simulink library "LibEEPROM_eeprom_example_ORIGINAL"  (Simulink 10.0)
settings: Solver=VariableStepAuto  StartTime=0.0  StopTime=10.0  RelTol=1e-3
undefined symbols (not defined in the file): CRC32_calc_and_EEPROM_Write_ALL, crc32_calc_intern, CRC32_EEPROM_Read, EEPROM_Mirror, EEPROM_Read, IO_Blk_Lib_TTC500, IO_EEPROM_GetStatus, IO_EEPROM_Init, IO_EEPROM_Write, Read_Mirror, Write_Mirror, Write_Mirror_prepare_EEPROM
libraries: simulink x56
(part 6 of 8)

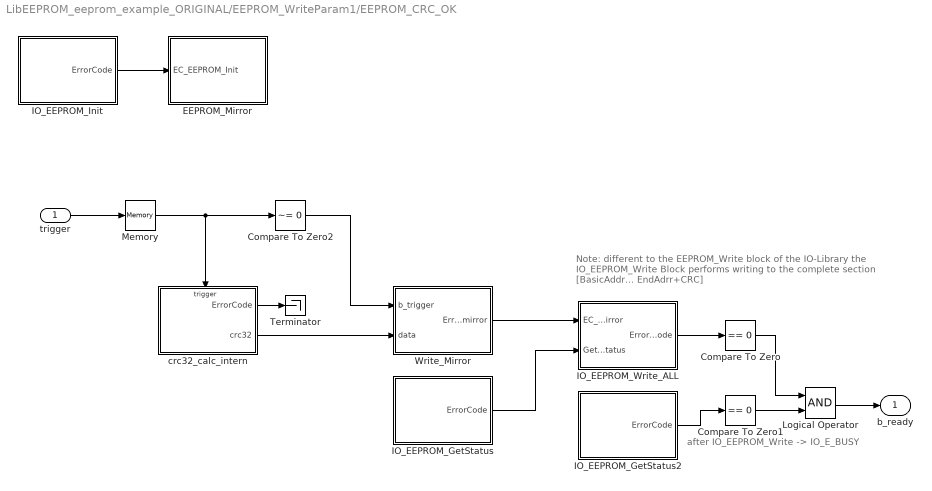
== system LibEEPROM_eeprom_example_ORIGINAL/EEPROM_WriteParam1/EEPROM_CRC_OK ==
  note: Note: different to the EEPROM_Write block
      | of the IO-Library the IO_EEPROM_Write Block
      | performs writing to the complete section [BasicAddr... EndAdrr+CRC]
  note: after IO_EEPROM_Write -> IO_E_BUSY
  trigger : Inport
  Compare To Zero : simulink/Logic and Bit Operations/Compare To Zero  relop===  OutDataTypeStr=boolean  ZeroCross=off
  Compare To Zero1 : simulink/Logic and Bit Operations/Compare To Zero  relop===  OutDataTypeStr=boolean  ZeroCross=off
  Compare To Zero2 : simulink/Logic and Bit Operations/Compare To Zero  relop=~=  OutDataTypeStr=boolean  ZeroCross=off
  EEPROM_Mirror : Subsystem  LoadFcn=|  mask(EEPROM_Mirror_Code){SampleTime=-1, ttlib=IO_Blk_Lib_TTC500, ttDescription=EEPROM_Mirror, tt_iolib_version=0.21, offset=0, length=65536}
      | try
      | %
      | %Upgrade Information - standard BEGIN
      | new_color = 'blue';
      | new_ver = '0.21';
      | act_ver = get_param(gcb,'tt_iolib_version');
      | if not(strcmp(act_ver,new_ver))
      |     disp(['Upgrade block: ',gcb,char(10),'       Version: ',act_ver,' -> ',new_ver]);
      |     %switch - case for specific upgrade information e.g. additional parameter required 
      |     %Change appearance and version information
      |     set_param(gcb,'ForegroundColor',new_color);
      |     set_param(gcb,'tt_iolib_version',new_ver);
      | end
      | %Upgrade Information - standard END
      | catch
      | %Standard catch section BEGIN 
      | disp(' ');
      | disp('------------------------------------------------------------');
      | disp('An error occurred in a callback of the TTC580-BlockLib.');
      | disp(['Please check the parameters in the mask of ',gcb]);
      | disp('If you do not encounter any violations, then please '); 
      | disp('copy the following lines and report this to support@ttcontrol.com ');
      | disp('<< begin of error message dump >>');
      | disp(['Version of TTC580-BlockLib: ', get_param(gcb,'tt_iolib_version')]);
      | disp(get_param(gcb,'ttDescription'));
      | disp(gcb);
      | x=lasterror;disp(x.message);
      | disp(get_param(gcb,'MaskValues'));
      | disp(version);
      | disp(computer);
      | disp('<< end of error message dump >>');
      | disp('------------------------------------------------------------');
      | disp(' ');
      | %Standard catch section END
      | end
      mask help:
      | Read all data from the EEPROM and mirror this onto RAM.
      | The ErrorCode of IO_EEPROM_Init - block must be connected to the input of EEPROM_Mirror.
      | After calling EEPROM_Mirror the global variable EEPROM_mirror is filled and
      | the global variable ErrorCode_EEPROM_mirror contains the returns of IO_EEPROM_Init() and IO_EEPROM_Read().
      mask init:
      | %
      settings: CopyFcn=%deleted
      mask Help: web(which('IO_EEPROM.h'))
      mask Callback offset: %
      mask Callback length: %
  IO_EEPROM_GetStatus : Subsystem  LoadFcn=|  mask(IO_EEPROM_GetStatus_Code){SampleTime=-1, ttlib=IO_Blk_Lib_TTC500, ttDescription=IO_EEPROM_GetStatus, tt_iolib_version=0.19}
      | try
      | %
      | %Upgrade Information - standard BEGIN
      | new_color = 'blue';
      | new_ver = '0.19';
      | act_ver = get_param(gcb,'tt_iolib_version');
      | if not(strcmp(act_ver,new_ver))
      |     disp(['Upgrade block: ',gcb,char(10),'       Version: ',act_ver,' -> ',new_ver]);
      |     %switch - case for specific upgrade information e.g. additional parameter required 
      |     %Change appearance and version information
      |     set_param(gcb,'ForegroundColor',new_color);
      |     set_param(gcb,'tt_iolib_version',new_ver);
      | end
      | %Upgrade Information - standard END
      | catch
      | %Standard catch section BEGIN 
      | disp(' ');
      | disp('------------------------------------------------------------');
      | disp('An error occurred in a callback of the TTC580-BlockLib.');
      | disp('Please copy the following lines and report this to support@tttech.com ');
      | disp('<< begin of error message dump >>');
      | disp(['Version of TTC580-BlockLib: ', get_param(gcb,'tt_iolib_version')]);
      | disp(get_param(gcb,'ttDescription'));
      | disp(gcb);
      | x=lasterror;disp(x.message);
      | disp(get_param(gcb,'MaskValues'));
      | disp(version);
      | disp(computer);
      | disp('<< end of error message dump >>');
      | disp('------------------------------------------------------------');
      | disp(' ');
      | %Standard catch section END
      | end
      mask help: Returns the status of the EEPROM driver.
      mask init:
      | %
      settings: CopyFcn=%deleted
      mask Help: web(which('IO_EEPROM.h'))
  IO_EEPROM_GetStatus2 : Subsystem  LoadFcn=|  mask(IO_EEPROM_GetStatus_Code){SampleTime=-1, ttlib=IO_Blk_Lib_TTC500, ttDescription=IO_EEPROM_GetStatus, tt_iolib_version=0.19}
      | try
      | %
      | %Upgrade Information - standard BEGIN
      | new_color = 'blue';
      | new_ver = '0.19';
      | act_ver = get_param(gcb,'tt_iolib_version');
      | if not(strcmp(act_ver,new_ver))
      |     disp(['Upgrade block: ',gcb,char(10),'       Version: ',act_ver,' -> ',new_ver]);
      |     %switch - case for specific upgrade information e.g. additional parameter required 
      |     %Change appearance and version information
      |     set_param(gcb,'ForegroundColor',new_color);
      |     set_param(gcb,'tt_iolib_version',new_ver);
      | end
      | %Upgrade Information - standard END
      | catch
      | %Standard catch section BEGIN 
      | disp(' ');
      | disp('------------------------------------------------------------');
      | disp('An error occurred in a callback of the TTC580-BlockLib.');
      | disp('Please copy the following lines and report this to support@tttech.com ');
      | disp('<< begin of error message dump >>');
      | disp(['Version of TTC580-BlockLib: ', get_param(gcb,'tt_iolib_version')]);
      | disp(get_param(gcb,'ttDescription'));
      | disp(gcb);
      | x=lasterror;disp(x.message);
      | disp(get_param(gcb,'MaskValues'));
      | disp(version);
      | disp(computer);
      | disp('<< end of error message dump >>');
      | disp('------------------------------------------------------------');
      | disp(' ');
      | %Standard catch section END
      | end
      mask help: Returns the status of the EEPROM driver.
      mask init:
      | %
      settings: CopyFcn=%deleted
      mask Help: web(which('IO_EEPROM.h'))
  IO_EEPROM_Init : Subsystem  LoadFcn=|  mask(IO_EEPROM_Init_Code){SampleTime=-1, ttlib=IO_Blk_Lib_TTC500, ttDescription=IO_EEPROM_Init, tt_iolib_version=0.19}
      | try
      | %
      | %Upgrade Information - standard BEGIN
      | new_color = 'blue';
      | new_ver = '0.19';
      | act_ver = get_param(gcb,'tt_iolib_version');
      | if not(strcmp(act_ver,new_ver))
      |     disp(['Upgrade block: ',gcb,char(10),'       Version: ',act_ver,' -> ',new_ver]);
      |     %switch - case for specific upgrade information e.g. additional parameter required 
      |     %Change appearance and version information
      |     set_param(gcb,'ForegroundColor',new_color);
      |     set_param(gcb,'tt_iolib_version',new_ver);
      | end
      | %Upgrade Information - standard END
      | catch
      | %Standard catch section BEGIN 
      | disp(' ');
      | disp('------------------------------------------------------------');
      | disp('An error occurred in a callback of the TTC580-BlockLib.');
      | disp('Please copy the following lines and report this to support@tttech.com ');
      | disp('<< begin of error message dump >>');
      | disp(['Version of TTC580-BlockLib: ', get_param(gcb,'tt_iolib_version')]);
      | disp(get_param(gcb,'ttDescription'));
      | disp(gcb);
      | x=lasterror;disp(x.message);
      | disp(get_param(gcb,'MaskValues'));
      | disp(version);
      | disp(computer);
      | disp('<< end of error message dump >>');
      | disp('------------------------------------------------------------');
      | disp(' ');
      | %Standard catch section END
      | end
      mask help: Initialization of the EEPROM driver.
      mask init:
      | %
      settings: CopyFcn=%deleted
      mask Help: web(which('IO_EEPROM.h'))
  IO_EEPROM_Write_ALL : Subsystem  LoadFcn=|  mask(IO_EEPROM_Write_Code){SampleTime=-1, ttlib=IO_Blk_Lib_TTC500, ttDescription=IO_EEPROM_Write, tt_iolib_version=0.19, offset=BasicAddr, length=EndAddr-BasicAddr+1+length}
      | try
      | %
      | %Upgrade Information - standard BEGIN
      | new_color = 'blue';
      | new_ver = '0.19';
      | act_ver = get_param(gcb,'tt_iolib_version');
      | if not(strcmp(act_ver,new_ver))
      |     disp(['Upgrade block: ',gcb,char(10),'       Version: ',act_ver,' -> ',new_ver]);
      |     %switch - case for specific upgrade information e.g. additional parameter required 
      |     %Change appearance and version information
      |     set_param(gcb,'ForegroundColor',new_color);
      |     set_param(gcb,'tt_iolib_version',new_ver);
      | end
      | %Upgrade Information - standard END
      | catch
      | %Standard catch section BEGIN 
      | disp(' ');
      | disp('------------------------------------------------------------');
      | disp('An error occurred in a callback of the TTC580-BlockLib.');
      | disp('Please copy the following lines and report this to support@tttech.com ');
      | disp('<< begin of error message dump >>');
      | disp(['Version of TTC580-BlockLib: ', get_param(gcb,'tt_iolib_version')]);
      | disp(get_param(gcb,'ttDescription'));
      | disp(gcb);
      | x=lasterror;disp(x.message);
      | disp(get_param(gcb,'MaskValues'));
      | disp(version);
      | disp(computer);
      | disp('<< end of error message dump >>');
      | disp('------------------------------------------------------------');
      | disp(' ');
      | %Standard catch section END
      | end
      mask help:
      | Copy data from EEPROM_mirror[] to physical EEPROM. Copy activity is triggered by the edge of the input "EC_Write_Mirror" from IO_E_BUSY to IO_E_OK.
      | The output "ErrorCode" is IO_E_BUSY as long as writing to EEPROM is pending. During the activities are performed writing to the physical EEPROM, "ErrorCode" corresponds to the output of the C-driver IO_EEPROM_Write().
      mask init:
      | %
      settings: CopyFcn=%deleted
      mask Help: web(which('IO_EEPROM.h'))
      mask Callback offset: %
      mask Callback length: %
  Logical Operator : Logic  AllPortsSameDT=off  OutDataTypeStr=boolean
  Memory : Memory  LinearizeAsDelay=on
  Terminator : Terminator
  Write_Mirror : Subsystem  LoadFcn=|  mask(Write_Mirror_Code){SampleTime=-1, ttlib=IO_Blk_Lib_TTC500, ttDescription=Write_Mirror, tt_iolib_version=0.19, offset=offset, length=length}
      | try
      | %
      | %Upgrade Information - standard BEGIN
      | new_color = 'blue';
      | new_ver = '0.19';
      | act_ver = get_param(gcb,'tt_iolib_version');
      | if not(strcmp(act_ver,new_ver))
      |     disp(['Upgrade block: ',gcb,char(10),'       Version: ',act_ver,' -> ',new_ver]);
      |     %switch - case for specific upgrade information e.g. additional parameter required 
      |     %Change appearance and version information
      |     set_param(gcb,'ForegroundColor',new_color);
      |     set_param(gcb,'tt_iolib_version',new_ver);
      | end
      | %Upgrade Information - standard END
      | catch
      | %Standard catch section BEGIN 
      | disp(' ');
      | disp('------------------------------------------------------------');
      | disp('An error occurred in a callback of the TTC580-BlockLib.');
      | disp('Please copy the following lines and report this to support@tttech.com ');
      | disp('<< begin of error message dump >>');
      | disp(['Version of TTC580-BlockLib: ', get_param(gcb,'tt_iolib_version')]);
      | disp(get_param(gcb,'ttDescription'));
      | disp(gcb);
      | x=lasterror;disp(x.message);
      | disp(get_param(gcb,'MaskValues'));
      | disp(version);
      | disp(computer);
      | disp('<< end of error message dump >>');
      | disp('------------------------------------------------------------');
      | disp(' ');
      | %Standard catch section END
      | end
      mask help:
      | Write data to the mirror of the EEPROM. ErrorCode is set to IO_E_BUSY for one cycle of writing into EEPROM_mirror[].
      | In case the given data section exceeds given EEPROM boundaries, IO_E_EEPROM_RANGE ErrorCode is returned.
      mask init:
      | %
      settings: CopyFcn=%deleted
      mask Help: web(which('~.h'))
      mask Callback offset: %
      mask Callback length: %
  crc32_calc_intern : Subsystem  LoadFcn=|  mask(crc32_calc_intern_Code){SampleTime=-1, ttlib=IO_Blk_Lib_TTC500, ttDescription=crc32_calc_intern, tt_iolib_version=0.19, EEPROM_mirror=EEPROM_mirror, iBasicAddr_intern=BasicAddr, iEndAddr_intern=EndAddr}
      | try
      | %
      | %Upgrade Information - standard BEGIN
      | new_color = 'blue';
      | new_ver = '0.19';
      | act_ver = get_param(gcb,'tt_iolib_version');
      | if not(strcmp(act_ver,new_ver))
      |     disp(['Upgrade block: ',gcb,char(10),'       Version: ',act_ver,' -> ',new_ver]);
      |     %switch - case for specific upgrade information e.g. additional parameter required 
      |     %Change appearance and version information
      |     set_param(gcb,'ForegroundColor',new_color);
      |     set_param(gcb,'tt_iolib_version',new_ver);
      | end
      | %Upgrade Information - standard END
      | catch
      | %Standard catch section BEGIN 
      | disp(' ');
      | disp('------------------------------------------------------------');
      | disp('An error occurred in a callback of the TTC580-BlockLib.');
      | disp('Please copy the following lines and report this to support@tttech.com ');
      | disp('<< begin of error message dump >>');
      | disp(['Version of TTC580-BlockLib: ', get_param(gcb,'tt_iolib_version')]);
      | disp(get_param(gcb,'ttDescription'));
      | disp(gcb);
      | x=lasterror;disp(x.message);
      | disp(get_param(gcb,'MaskValues'));
      | disp(version);
      | disp(computer);
      | disp('<< end of error message dump >>');
      | disp('------------------------------------------------------------');
      | disp(' ');
      | %Standard catch section END
      | end
      mask help:
      | Calculate crc32 for a section out of the EEPROM.
      | In case the given data section exceeds given EEPROM boundaries, non zero ErrorCode is returned.
      mask init:
      | %
      settings: CopyFcn=%deleted
      mask Help: No further help available for this block
      mask Callback EEPROM_mirror: %
      mask Callback iBasicAddr_intern: %
      mask Callback iEndAddr_intern: %
  b_ready : Outport  VectorParamsAs1DForOutWhenUnconnected=off
  wires:
  Compare To Zero1/1 -> Logical Operator/2
  crc32_calc_intern/1(ErrorCode) -> Terminator/1
  Logical Operator/1 -> b_ready/1
  Compare To Zero/1 -> Logical Operator/1
  Memory/1 -> Compare To Zero2/1, crc32_calc_intern/Trigger
  Compare To Zero2/1 -> Write_Mirror/1(b_trigger)
  crc32_calc_intern/2(crc32) -> Write_Mirror/2(data)
  IO_EEPROM_GetStatus/1(ErrorCode) -> IO_EEPROM_Write_ALL/2(GetStatus)
  Write_Mirror/1(ErrorCode_EEPROM_mirror) -> IO_EEPROM_Write_ALL/1(EC_Write_Mirror)
  trigger/1 -> Memory/1
  IO_EEPROM_Write_ALL/1(ErrorCode) -> Compare To Zero/1
  IO_EEPROM_Init/1(ErrorCode) -> EEPROM_Mirror/1(EC_EEPROM_Init)
  IO_EEPROM_GetStatus2/1(ErrorCode) -> Compare To Zero1/1

== system LibEEPROM_eeprom_example_ORIGINAL/EEPROM_WriteParam1/EEPROM_param_1 ==
  note: NO IO_EEPROM_Write
      | perfomted here. This is
      | done in CRC32_calc_and_EEPROM_Write_ALL
  trigger : Inport
  data : Inport  Port=2  OutDataTypeStr=EEPROM_type
  Compare To Zero : simulink/Logic and Bit Operations/Compare To Zero  relop===  OutDataTypeStr=boolean  ZeroCross=off
  Compare To Zero1 : simulink/Logic and Bit Operations/Compare To Zero  relop=~=  OutDataTypeStr=boolean  ZeroCross=off
  Write_Mirror : Subsystem  LoadFcn=|  mask(Write_Mirror_Code){SampleTime=-1, ttlib=IO_Blk_Lib_TTC500, ttDescription=Write_Mirror, tt_iolib_version=0.19, offset=offset, length=length}
      | try
      | %
      | %Upgrade Information - standard BEGIN
      | new_color = 'blue';
      | new_ver = '0.19';
      | act_ver = get_param(gcb,'tt_iolib_version');
      | if not(strcmp(act_ver,new_ver))
      |     disp(['Upgrade block: ',gcb,char(10),'       Version: ',act_ver,' -> ',new_ver]);
      |     %switch - case for specific upgrade information e.g. additional parameter required 
      |     %Change appearance and version information
      |     set_param(gcb,'ForegroundColor',new_color);
      |     set_param(gcb,'tt_iolib_version',new_ver);
      | end
      | %Upgrade Information - standard END
      | catch
      | %Standard catch section BEGIN 
      | disp(' ');
      | disp('------------------------------------------------------------');
      | disp('An error occurred in a callback of the TTC580-BlockLib.');
      | disp('Please copy the following lines and report this to support@tttech.com ');
      | disp('<< begin of error message dump >>');
      | disp(['Version of TTC580-BlockLib: ', get_param(gcb,'tt_iolib_version')]);
      | disp(get_param(gcb,'ttDescription'));
      | disp(gcb);
      | x=lasterror;disp(x.message);
      | disp(get_param(gcb,'MaskValues'));
      | disp(version);
      | disp(computer);
      | disp('<< end of error message dump >>');
      | disp('------------------------------------------------------------');
      | disp(' ');
      | %Standard catch section END
      | end
      mask help:
      | Write data to the mirror of the EEPROM. ErrorCode is set to IO_E_BUSY for one cycle of writing into EEPROM_mirror[].
      | In case the given data section exceeds given EEPROM boundaries, IO_E_EEPROM_RANGE ErrorCode is returned.
      mask init:
      | %
      settings: CopyFcn=%deleted
      mask Help: web(which('~.h'))
      mask Callback offset: %
      mask Callback length: %
  b_ready : Outport  VectorParamsAs1DForOutWhenUnconnected=off
  wires:
  Compare To Zero1/1 -> Write_Mirror/1(b_trigger)
  Write_Mirror/1(ErrorCode_EEPROM_mirror) -> Compare To Zero/1
  data/1 -> Write_Mirror/2(data)
  trigger/1 -> Compare To Zero1/1
  Compare To Zero/1 -> b_ready/1

== system LibEEPROM_eeprom_example_ORIGINAL/EEPROM_WriteParam1/EEPROM_param_2 ==
  note: NO IO_EEPROM_Write
      | perfomted here. This is
      | done in CRC32_calc_and_EEPROM_Write_ALL
  trigger : Inport
  data : Inport  Port=2  OutDataTypeStr=EEPROM_type
  Compare To Zero : simulink/Logic and Bit Operations/Compare To Zero  relop===  OutDataTypeStr=boolean  ZeroCross=off
  Compare To Zero1 : simulink/Logic and Bit Operations/Compare To Zero  relop=~=  OutDataTypeStr=boolean  ZeroCross=off
  Write_Mirror : Subsystem  LoadFcn=|  mask(Write_Mirror_Code){SampleTime=-1, ttlib=IO_Blk_Lib_TTC500, ttDescription=Write_Mirror, tt_iolib_version=0.19, offset=offset, length=length}
      | try
      | %
      | %Upgrade Information - standard BEGIN
      | new_color = 'blue';
      | new_ver = '0.19';
      | act_ver = get_param(gcb,'tt_iolib_version');
      | if not(strcmp(act_ver,new_ver))
      |     disp(['Upgrade block: ',gcb,char(10),'       Version: ',act_ver,' -> ',new_ver]);
      |     %switch - case for specific upgrade information e.g. additional parameter required 
      |     %Change appearance and version information
      |     set_param(gcb,'ForegroundColor',new_color);
      |     set_param(gcb,'tt_iolib_version',new_ver);
      | end
      | %Upgrade Information - standard END
      | catch
      | %Standard catch section BEGIN 
      | disp(' ');
      | disp('------------------------------------------------------------');
      | disp('An error occurred in a callback of the TTC580-BlockLib.');
      | disp('Please copy the following lines and report this to support@tttech.com ');
      | disp('<< begin of error message dump >>');
      | disp(['Version of TTC580-BlockLib: ', get_param(gcb,'tt_iolib_version')]);
      | disp(get_param(gcb,'ttDescription'));
      | disp(gcb);
      | x=lasterror;disp(x.message);
      | disp(get_param(gcb,'MaskValues'));
      | disp(version);
      | disp(computer);
      | disp('<< end of error message dump >>');
      | disp('------------------------------------------------------------');
      | disp(' ');
      | %Standard catch section END
      | end
      mask help:
      | Write data to the mirror of the EEPROM. ErrorCode is set to IO_E_BUSY for one cycle of writing into EEPROM_mirror[].
      | In case the given data section exceeds given EEPROM boundaries, IO_E_EEPROM_RANGE ErrorCode is returned.
      mask init:
      | %
      settings: CopyFcn=%deleted
      mask Help: web(which('~.h'))
      mask Callback offset: %
      mask Callback length: %
  b_ready : Outport  VectorParamsAs1DForOutWhenUnconnected=off
  wires:
  Compare To Zero1/1 -> Write_Mirror/1(b_trigger)
  Write_Mirror/1(ErrorCode_EEPROM_mirror) -> Compare To Zero/1
  data/1 -> Write_Mirror/2(data)
  trigger/1 -> Compare To Zero1/1
  Compare To Zero/1 -> b_ready/1

== system LibEEPROM_eeprom_example_ORIGINAL/EEPROM_WriteParam1/EEPROM_param_3 ==
  note: NO IO_EEPROM_Write
      | perfomted here. This is
      | done in CRC32_calc_and_EEPROM_Write_ALL
  trigger : Inport
  data : Inport  Port=2  OutDataTypeStr=EEPROM_type
  Compare To Zero : simulink/Logic and Bit Operations/Compare To Zero  relop===  OutDataTypeStr=boolean  ZeroCross=off
  Compare To Zero1 : simulink/Logic and Bit Operations/Compare To Zero  relop=~=  OutDataTypeStr=boolean  ZeroCross=off
  Write_Mirror : Subsystem  LoadFcn=|  mask(Write_Mirror_Code){SampleTime=-1, ttlib=IO_Blk_Lib_TTC500, ttDescription=Write_Mirror, tt_iolib_version=0.19, offset=offset, length=length}
      | try
      | %
      | %Upgrade Information - standard BEGIN
      | new_color = 'blue';
      | new_ver = '0.19';
      | act_ver = get_param(gcb,'tt_iolib_version');
      | if not(strcmp(act_ver,new_ver))
      |     disp(['Upgrade block: ',gcb,char(10),'       Version: ',act_ver,' -> ',new_ver]);
      |     %switch - case for specific upgrade information e.g. additional parameter required 
      |     %Change appearance and version information
      |     set_param(gcb,'ForegroundColor',new_color);
      |     set_param(gcb,'tt_iolib_version',new_ver);
      | end
      | %Upgrade Information - standard END
      | catch
      | %Standard catch section BEGIN 
      | disp(' ');
      | disp('------------------------------------------------------------');
      | disp('An error occurred in a callback of the TTC580-BlockLib.');
      | disp('Please copy the following lines and report this to support@tttech.com ');
      | disp('<< begin of error message dump >>');
      | disp(['Version of TTC580-BlockLib: ', get_param(gcb,'tt_iolib_version')]);
      | disp(get_param(gcb,'ttDescription'));
      | disp(gcb);
      | x=lasterror;disp(x.message);
      | disp(get_param(gcb,'MaskValues'));
      | disp(version);
      | disp(computer);
      | disp('<< end of error message dump >>');
      | disp('------------------------------------------------------------');
      | disp(' ');
      | %Standard catch section END
      | end
      mask help:
      | Write data to the mirror of the EEPROM. ErrorCode is set to IO_E_BUSY for one cycle of writing into EEPROM_mirror[].
      | In case the given data section exceeds given EEPROM boundaries, IO_E_EEPROM_RANGE ErrorCode is returned.
      mask init:
      | %
      settings: CopyFcn=%deleted
      mask Help: web(which('~.h'))
      mask Callback offset: %
      mask Callback length: %
  b_ready : Outport  VectorParamsAs1DForOutWhenUnconnected=off
  wires:
  Compare To Zero1/1 -> Write_Mirror/1(b_trigger)
  Write_Mirror/1(ErrorCode_EEPROM_mirror) -> Compare To Zero/1
  data/1 -> Write_Mirror/2(data)
  trigger/1 -> Compare To Zero1/1
  Compare To Zero/1 -> b_ready/1

== system LibEEPROM_eeprom_example_ORIGINAL/EEPROM_WriteParam1/EEPROM_param_4 ==
  note: NO IO_EEPROM_Write
      | perfomted here. This is
      | done in CRC32_calc_and_EEPROM_Write_ALL
  trigger : Inport
  data : Inport  Port=2  OutDataTypeStr=EEPROM_type
  Compare To Zero : simulink/Logic and Bit Operations/Compare To Zero  relop===  OutDataTypeStr=boolean  ZeroCross=off
  Compare To Zero1 : simulink/Logic and Bit Operations/Compare To Zero  relop=~=  OutDataTypeStr=boolean  ZeroCross=off
  Write_Mirror : Subsystem  LoadFcn=|  mask(Write_Mirror_Code){SampleTime=-1, ttlib=IO_Blk_Lib_TTC500, ttDescription=Write_Mirror, tt_iolib_version=0.19, offset=offset, length=length}
      | try
      | %
      | %Upgrade Information - standard BEGIN
      | new_color = 'blue';
      | new_ver = '0.19';
      | act_ver = get_param(gcb,'tt_iolib_version');
      | if not(strcmp(act_ver,new_ver))
      |     disp(['Upgrade block: ',gcb,char(10),'       Version: ',act_ver,' -> ',new_ver]);
      |     %switch - case for specific upgrade information e.g. additional parameter required 
      |     %Change appearance and version information
      |     set_param(gcb,'ForegroundColor',new_color);
      |     set_param(gcb,'tt_iolib_version',new_ver);
      | end
      | %Upgrade Information - standard END
      | catch
      | %Standard catch section BEGIN 
      | disp(' ');
      | disp('------------------------------------------------------------');
      | disp('An error occurred in a callback of the TTC580-BlockLib.');
      | disp('Please copy the following lines and report this to support@tttech.com ');
      | disp('<< begin of error message dump >>');
      | disp(['Version of TTC580-BlockLib: ', get_param(gcb,'tt_iolib_version')]);
      | disp(get_param(gcb,'ttDescription'));
      | disp(gcb);
      | x=lasterror;disp(x.message);
      | disp(get_param(gcb,'MaskValues'));
      | disp(version);
      | disp(computer);
      | disp('<< end of error message dump >>');
      | disp('------------------------------------------------------------');
      | disp(' ');
      | %Standard catch section END
      | end
      mask help:
      | Write data to the mirror of the EEPROM. ErrorCode is set to IO_E_BUSY for one cycle of writing into EEPROM_mirror[].
      | In case the given data section exceeds given EEPROM boundaries, IO_E_EEPROM_RANGE ErrorCode is returned.
      mask init:
      | %
      settings: CopyFcn=%deleted
      mask Help: web(which('~.h'))
      mask Callback offset: %
      mask Callback length: %
  b_ready : Outport  VectorParamsAs1DForOutWhenUnconnected=off
  wires:
  Compare To Zero1/1 -> Write_Mirror/1(b_trigger)
  Write_Mirror/1(ErrorCode_EEPROM_mirror) -> Compare To Zero/1
  data/1 -> Write_Mirror/2(data)
  trigger/1 -> Compare To Zero1/1
  Compare To Zero/1 -> b_ready/1

== system LibEEPROM_eeprom_example_ORIGINAL/EEPROM_WriteParam1/EEPROM_param_5 ==
  note: NO IO_EEPROM_Write
      | perfomted here. This is
      | done in CRC32_calc_and_EEPROM_Write_ALL
  trigger : Inport
  data : Inport  Port=2  OutDataTypeStr=EEPROM_type
  Compare To Zero : simulink/Logic and Bit Operations/Compare To Zero  relop===  OutDataTypeStr=boolean  ZeroCross=off
  Compare To Zero1 : simulink/Logic and Bit Operations/Compare To Zero  relop=~=  OutDataTypeStr=boolean  ZeroCross=off
  Write_Mirror : Subsystem  LoadFcn=|  mask(Write_Mirror_Code){SampleTime=-1, ttlib=IO_Blk_Lib_TTC500, ttDescription=Write_Mirror, tt_iolib_version=0.19, offset=offset, length=length}
      | try
      | %
      | %Upgrade Information - standard BEGIN
      | new_color = 'blue';
      | new_ver = '0.19';
      | act_ver = get_param(gcb,'tt_iolib_version');
      | if not(strcmp(act_ver,new_ver))
      |     disp(['Upgrade block: ',gcb,char(10),'       Version: ',act_ver,' -> ',new_ver]);
      |     %switch - case for specific upgrade information e.g. additional parameter required 
      |     %Change appearance and version information
      |     set_param(gcb,'ForegroundColor',new_color);
      |     set_param(gcb,'tt_iolib_version',new_ver);
      | end
      | %Upgrade Information - standard END
      | catch
      | %Standard catch section BEGIN 
      | disp(' ');
      | disp('------------------------------------------------------------');
      | disp('An error occurred in a callback of the TTC580-BlockLib.');
      | disp('Please copy the following lines and report this to support@tttech.com ');
      | disp('<< begin of error message dump >>');
      | disp(['Version of TTC580-BlockLib: ', get_param(gcb,'tt_iolib_version')]);
      | disp(get_param(gcb,'ttDescription'));
      | disp(gcb);
      | x=lasterror;disp(x.message);
      | disp(get_param(gcb,'MaskValues'));
      | disp(version);
      | disp(computer);
      | disp('<< end of error message dump >>');
      | disp('------------------------------------------------------------');
      | disp(' ');
      | %Standard catch section END
      | end
      mask help:
      | Write data to the mirror of the EEPROM. ErrorCode is set to IO_E_BUSY for one cycle of writing into EEPROM_mirror[].
      | In case the given data section exceeds given EEPROM boundaries, IO_E_EEPROM_RANGE ErrorCode is returned.
      mask init:
      | %
      settings: CopyFcn=%deleted
      mask Help: web(which('~.h'))
      mask Callback offset: %
      mask Callback length: %
  b_ready : Outport  VectorParamsAs1DForOutWhenUnconnected=off
  wires:
  Compare To Zero1/1 -> Write_Mirror/1(b_trigger)
  Write_Mirror/1(ErrorCode_EEPROM_mirror) -> Compare To Zero/1
  data/1 -> Write_Mirror/2(data)
  trigger/1 -> Compare To Zero1/1
  Compare To Zero/1 -> b_ready/1

== system LibEEPROM_eeprom_example_ORIGINAL/EEPROM_WriteParam1/EEPROM_param_6 ==
  note: NO IO_EEPROM_Write
      | perfomted here. This is
      | done in CRC32_calc_and_EEPROM_Write_ALL
  trigger : Inport
  data : Inport  Port=2  OutDataTypeStr=EEPROM_type
  Compare To Zero : simulink/Logic and Bit Operations/Compare To Zero  relop===  OutDataTypeStr=boolean  ZeroCross=off
  Compare To Zero1 : simulink/Logic and Bit Operations/Compare To Zero  relop=~=  OutDataTypeStr=boolean  ZeroCross=off
  Write_Mirror : Subsystem  LoadFcn=|  mask(Write_Mirror_Code){SampleTime=-1, ttlib=IO_Blk_Lib_TTC500, ttDescription=Write_Mirror, tt_iolib_version=0.19, offset=offset, length=length}
      | try
      | %
      | %Upgrade Information - standard BEGIN
      | new_color = 'blue';
      | new_ver = '0.19';
      | act_ver = get_param(gcb,'tt_iolib_version');
      | if not(strcmp(act_ver,new_ver))
      |     disp(['Upgrade block: ',gcb,char(10),'       Version: ',act_ver,' -> ',new_ver]);
      |     %switch - case for specific upgrade information e.g. additional parameter required 
      |     %Change appearance and version information
      |     set_param(gcb,'ForegroundColor',new_color);
      |     set_param(gcb,'tt_iolib_version',new_ver);
      | end
      | %Upgrade Information - standard END
      | catch
      | %Standard catch section BEGIN 
      | disp(' ');
      | disp('------------------------------------------------------------');
      | disp('An error occurred in a callback of the TTC580-BlockLib.');
      | disp('Please copy the following lines and report this to support@tttech.com ');
      | disp('<< begin of error message dump >>');
      | disp(['Version of TTC580-BlockLib: ', get_param(gcb,'tt_iolib_version')]);
      | disp(get_param(gcb,'ttDescription'));
      | disp(gcb);
      | x=lasterror;disp(x.message);
      | disp(get_param(gcb,'MaskValues'));
      | disp(version);
      | disp(computer);
      | disp('<< end of error message dump >>');
      | disp('------------------------------------------------------------');
      | disp(' ');
      | %Standard catch section END
      | end
      mask help:
      | Write data to the mirror of the EEPROM. ErrorCode is set to IO_E_BUSY for one cycle of writing into EEPROM_mirror[].
      | In case the given data section exceeds given EEPROM boundaries, IO_E_EEPROM_RANGE ErrorCode is returned.
      mask init:
      | %
      settings: CopyFcn=%deleted
      mask Help: web(which('~.h'))
      mask Callback offset: %
      mask Callback length: %
  b_ready : Outport  VectorParamsAs1DForOutWhenUnconnected=off
  wires:
  Compare To Zero1/1 -> Write_Mirror/1(b_trigger)
  Write_Mirror/1(ErrorCode_EEPROM_mirror) -> Compare To Zero/1
  data/1 -> Write_Mirror/2(data)
  trigger/1 -> Compare To Zero1/1
  Compare To Zero/1 -> b_ready/1

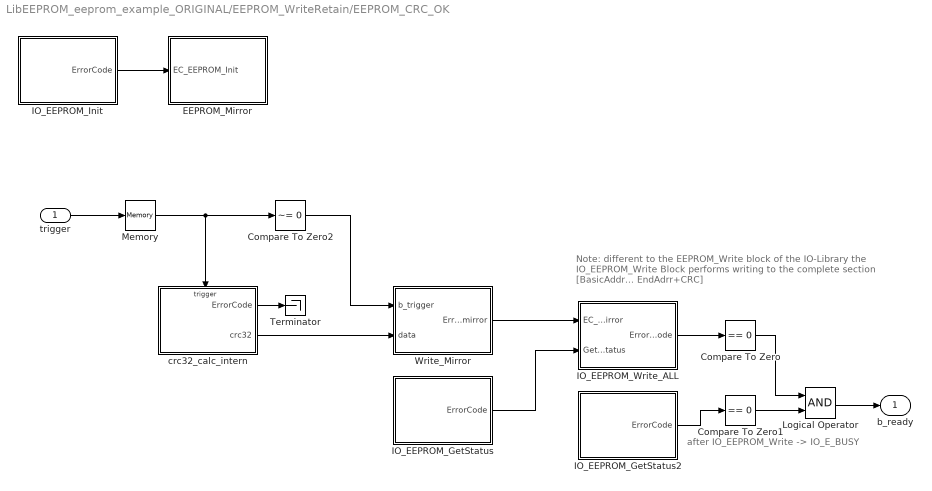
== system LibEEPROM_eeprom_example_ORIGINAL/EEPROM_WriteRetain/EEPROM_CRC_OK ==
  note: Note: different to the EEPROM_Write block
      | of the IO-Library the IO_EEPROM_Write Block
      | performs writing to the complete section [BasicAddr... EndAdrr+CRC]
  note: after IO_EEPROM_Write -> IO_E_BUSY
  trigger : Inport
  Compare To Zero : simulink/Logic and Bit Operations/Compare To Zero  relop===  OutDataTypeStr=boolean  ZeroCross=off
  Compare To Zero1 : simulink/Logic and Bit Operations/Compare To Zero  relop===  OutDataTypeStr=boolean  ZeroCross=off
  Compare To Zero2 : simulink/Logic and Bit Operations/Compare To Zero  relop=~=  OutDataTypeStr=boolean  ZeroCross=off
  EEPROM_Mirror : Subsystem  LoadFcn=|  mask(EEPROM_Mirror_Code){SampleTime=-1, ttlib=IO_Blk_Lib_TTC500, ttDescription=EEPROM_Mirror, tt_iolib_version=0.21, offset=0, length=65536}
      | try
      | %
      | %Upgrade Information - standard BEGIN
      | new_color = 'blue';
      | new_ver = '0.21';
      | act_ver = get_param(gcb,'tt_iolib_version');
      | if not(strcmp(act_ver,new_ver))
      |     disp(['Upgrade block: ',gcb,char(10),'       Version: ',act_ver,' -> ',new_ver]);
      |     %switch - case for specific upgrade information e.g. additional parameter required 
      |     %Change appearance and version information
      |     set_param(gcb,'ForegroundColor',new_color);
      |     set_param(gcb,'tt_iolib_version',new_ver);
      | end
      | %Upgrade Information - standard END
      | catch
      | %Standard catch section BEGIN 
      | disp(' ');
      | disp('------------------------------------------------------------');
      | disp('An error occurred in a callback of the TTC580-BlockLib.');
      | disp(['Please check the parameters in the mask of ',gcb]);
      | disp('If you do not encounter any violations, then please '); 
      | disp('copy the following lines and report this to support@ttcontrol.com ');
      | disp('<< begin of error message dump >>');
      | disp(['Version of TTC580-BlockLib: ', get_param(gcb,'tt_iolib_version')]);
      | disp(get_param(gcb,'ttDescription'));
      | disp(gcb);
      | x=lasterror;disp(x.message);
      | disp(get_param(gcb,'MaskValues'));
      | disp(version);
      | disp(computer);
      | disp('<< end of error message dump >>');
      | disp('------------------------------------------------------------');
      | disp(' ');
      | %Standard catch section END
      | end
      mask help:
      | Read all data from the EEPROM and mirror this onto RAM.
      | The ErrorCode of IO_EEPROM_Init - block must be connected to the input of EEPROM_Mirror.
      | After calling EEPROM_Mirror the global variable EEPROM_mirror is filled and
      | the global variable ErrorCode_EEPROM_mirror contains the returns of IO_EEPROM_Init() and IO_EEPROM_Read().
      mask init:
      | %
      settings: CopyFcn=%deleted
      mask Help: web(which('IO_EEPROM.h'))
      mask Callback offset: %
      mask Callback length: %
  IO_EEPROM_GetStatus : Subsystem  LoadFcn=|  mask(IO_EEPROM_GetStatus_Code){SampleTime=-1, ttlib=IO_Blk_Lib_TTC500, ttDescription=IO_EEPROM_GetStatus, tt_iolib_version=0.19}
      | try
      | %
      | %Upgrade Information - standard BEGIN
      | new_color = 'blue';
      | new_ver = '0.19';
      | act_ver = get_param(gcb,'tt_iolib_version');
      | if not(strcmp(act_ver,new_ver))
      |     disp(['Upgrade block: ',gcb,char(10),'       Version: ',act_ver,' -> ',new_ver]);
      |     %switch - case for specific upgrade information e.g. additional parameter required 
      |     %Change appearance and version information
      |     set_param(gcb,'ForegroundColor',new_color);
      |     set_param(gcb,'tt_iolib_version',new_ver);
      | end
      | %Upgrade Information - standard END
      | catch
      | %Standard catch section BEGIN 
      | disp(' ');
      | disp('------------------------------------------------------------');
      | disp('An error occurred in a callback of the TTC580-BlockLib.');
      | disp('Please copy the following lines and report this to support@tttech.com ');
      | disp('<< begin of error message dump >>');
      | disp(['Version of TTC580-BlockLib: ', get_param(gcb,'tt_iolib_version')]);
      | disp(get_param(gcb,'ttDescription'));
      | disp(gcb);
      | x=lasterror;disp(x.message);
      | disp(get_param(gcb,'MaskValues'));
      | disp(version);
      | disp(computer);
      | disp('<< end of error message dump >>');
      | disp('------------------------------------------------------------');
      | disp(' ');
      | %Standard catch section END
      | end
      mask help: Returns the status of the EEPROM driver.
      mask init:
      | %
      settings: CopyFcn=%deleted
      mask Help: web(which('IO_EEPROM.h'))
  IO_EEPROM_GetStatus2 : Subsystem  LoadFcn=|  mask(IO_EEPROM_GetStatus_Code){SampleTime=-1, ttlib=IO_Blk_Lib_TTC500, ttDescription=IO_EEPROM_GetStatus, tt_iolib_version=0.19}
      | try
      | %
      | %Upgrade Information - standard BEGIN
      | new_color = 'blue';
      | new_ver = '0.19';
      | act_ver = get_param(gcb,'tt_iolib_version');
      | if not(strcmp(act_ver,new_ver))
      |     disp(['Upgrade block: ',gcb,char(10),'       Version: ',act_ver,' -> ',new_ver]);
      |     %switch - case for specific upgrade information e.g. additional parameter required 
      |     %Change appearance and version information
      |     set_param(gcb,'ForegroundColor',new_color);
      |     set_param(gcb,'tt_iolib_version',new_ver);
      | end
      | %Upgrade Information - standard END
      | catch
      | %Standard catch section BEGIN 
      | disp(' ');
      | disp('------------------------------------------------------------');
      | disp('An error occurred in a callback of the TTC580-BlockLib.');
      | disp('Please copy the following lines and report this to support@tttech.com ');
      | disp('<< begin of error message dump >>');
      | disp(['Version of TTC580-BlockLib: ', get_param(gcb,'tt_iolib_version')]);
      | disp(get_param(gcb,'ttDescription'));
      | disp(gcb);
      | x=lasterror;disp(x.message);
      | disp(get_param(gcb,'MaskValues'));
      | disp(version);
      | disp(computer);
      | disp('<< end of error message dump >>');
      | disp('------------------------------------------------------------');
      | disp(' ');
      | %Standard catch section END
      | end
      mask help: Returns the status of the EEPROM driver.
      mask init:
      | %
      settings: CopyFcn=%deleted
      mask Help: web(which('IO_EEPROM.h'))
  IO_EEPROM_Init : Subsystem  LoadFcn=|  mask(IO_EEPROM_Init_Code){SampleTime=-1, ttlib=IO_Blk_Lib_TTC500, ttDescription=IO_EEPROM_Init, tt_iolib_version=0.19}
      | try
      | %
      | %Upgrade Information - standard BEGIN
      | new_color = 'blue';
      | new_ver = '0.19';
      | act_ver = get_param(gcb,'tt_iolib_version');
      | if not(strcmp(act_ver,new_ver))
      |     disp(['Upgrade block: ',gcb,char(10),'       Version: ',act_ver,' -> ',new_ver]);
      |     %switch - case for specific upgrade information e.g. additional parameter required 
      |     %Change appearance and version information
      |     set_param(gcb,'ForegroundColor',new_color);
      |     set_param(gcb,'tt_iolib_version',new_ver);
      | end
      | %Upgrade Information - standard END
      | catch
      | %Standard catch section BEGIN 
      | disp(' ');
      | disp('------------------------------------------------------------');
      | disp('An error occurred in a callback of the TTC580-BlockLib.');
      | disp('Please copy the following lines and report this to support@tttech.com ');
      | disp('<< begin of error message dump >>');
      | disp(['Version of TTC580-BlockLib: ', get_param(gcb,'tt_iolib_version')]);
      | disp(get_param(gcb,'ttDescription'));
      | disp(gcb);
      | x=lasterror;disp(x.message);
      | disp(get_param(gcb,'MaskValues'));
      | disp(version);
      | disp(computer);
      | disp('<< end of error message dump >>');
      | disp('------------------------------------------------------------');
      | disp(' ');
      | %Standard catch section END
      | end
      mask help: Initialization of the EEPROM driver.
      mask init:
      | %
      settings: CopyFcn=%deleted
      mask Help: web(which('IO_EEPROM.h'))
  IO_EEPROM_Write_ALL : Subsystem  LoadFcn=|  mask(IO_EEPROM_Write_Code){SampleTime=-1, ttlib=IO_Blk_Lib_TTC500, ttDescription=IO_EEPROM_Write, tt_iolib_version=0.19, offset=BasicAddr, length=EndAddr-BasicAddr+1+length}
      | try
      | %
      | %Upgrade Information - standard BEGIN
      | new_color = 'blue';
      | new_ver = '0.19';
      | act_ver = get_param(gcb,'tt_iolib_version');
      | if not(strcmp(act_ver,new_ver))
      |     disp(['Upgrade block: ',gcb,char(10),'       Version: ',act_ver,' -> ',new_ver]);
      |     %switch - case for specific upgrade information e.g. additional parameter required 
      |     %Change appearance and version information
      |     set_param(gcb,'ForegroundColor',new_color);
      |     set_param(gcb,'tt_iolib_version',new_ver);
      | end
      | %Upgrade Information - standard END
      | catch
      | %Standard catch section BEGIN 
      | disp(' ');
      | disp('------------------------------------------------------------');
      | disp('An error occurred in a callback of the TTC580-BlockLib.');
      | disp('Please copy the following lines and report this to support@tttech.com ');
      | disp('<< begin of error message dump >>');
      | disp(['Version of TTC580-BlockLib: ', get_param(gcb,'tt_iolib_version')]);
      | disp(get_param(gcb,'ttDescription'));
      | disp(gcb);
      | x=lasterror;disp(x.message);
      | disp(get_param(gcb,'MaskValues'));
      | disp(version);
      | disp(computer);
      | disp('<< end of error message dump >>');
      | disp('------------------------------------------------------------');
      | disp(' ');
      | %Standard catch section END
      | end
      mask help:
      | Copy data from EEPROM_mirror[] to physical EEPROM. Copy activity is triggered by the edge of the input "EC_Write_Mirror" from IO_E_BUSY to IO_E_OK.
      | The output "ErrorCode" is IO_E_BUSY as long as writing to EEPROM is pending. During the activities are performed writing to the physical EEPROM, "ErrorCode" corresponds to the output of the C-driver IO_EEPROM_Write().
      mask init:
      | %
      settings: CopyFcn=%deleted
      mask Help: web(which('IO_EEPROM.h'))
      mask Callback offset: %
      mask Callback length: %
  Logical Operator : Logic  AllPortsSameDT=off  OutDataTypeStr=boolean
  Memory : Memory  LinearizeAsDelay=on
  Terminator : Terminator
  Write_Mirror : Subsystem  LoadFcn=|  mask(Write_Mirror_Code){SampleTime=-1, ttlib=IO_Blk_Lib_TTC500, ttDescription=Write_Mirror, tt_iolib_version=0.19, offset=offset, length=length}
      | try
      | %
      | %Upgrade Information - standard BEGIN
      | new_color = 'blue';
      | new_ver = '0.19';
      | act_ver = get_param(gcb,'tt_iolib_version');
      | if not(strcmp(act_ver,new_ver))
      |     disp(['Upgrade block: ',gcb,char(10),'       Version: ',act_ver,' -> ',new_ver]);
      |     %switch - case for specific upgrade information e.g. additional parameter required 
      |     %Change appearance and version information
      |     set_param(gcb,'ForegroundColor',new_color);
      |     set_param(gcb,'tt_iolib_version',new_ver);
      | end
      | %Upgrade Information - standard END
      | catch
      | %Standard catch section BEGIN 
      | disp(' ');
      | disp('------------------------------------------------------------');
      | disp('An error occurred in a callback of the TTC580-BlockLib.');
      | disp('Please copy the following lines and report this to support@tttech.com ');
      | disp('<< begin of error message dump >>');
      | disp(['Version of TTC580-BlockLib: ', get_param(gcb,'tt_iolib_version')]);
      | disp(get_param(gcb,'ttDescription'));
      | disp(gcb);
      | x=lasterror;disp(x.message);
      | disp(get_param(gcb,'MaskValues'));
      | disp(version);
      | disp(computer);
      | disp('<< end of error message dump >>');
      | disp('------------------------------------------------------------');
      | disp(' ');
      | %Standard catch section END
      | end
      mask help:
      | Write data to the mirror of the EEPROM. ErrorCode is set to IO_E_BUSY for one cycle of writing into EEPROM_mirror[].
      | In case the given data section exceeds given EEPROM boundaries, IO_E_EEPROM_RANGE ErrorCode is returned.
      mask init:
      | %
      settings: CopyFcn=%deleted
      mask Help: web(which('~.h'))
      mask Callback offset: %
      mask Callback length: %
  crc32_calc_intern : Subsystem  LoadFcn=|  mask(crc32_calc_intern_Code){SampleTime=-1, ttlib=IO_Blk_Lib_TTC500, ttDescription=crc32_calc_intern, tt_iolib_version=0.19, EEPROM_mirror=EEPROM_mirror, iBasicAddr_intern=BasicAddr, iEndAddr_intern=EndAddr}
      | try
      | %
      | %Upgrade Information - standard BEGIN
      | new_color = 'blue';
      | new_ver = '0.19';
      | act_ver = get_param(gcb,'tt_iolib_version');
      | if not(strcmp(act_ver,new_ver))
      |     disp(['Upgrade block: ',gcb,char(10),'       Version: ',act_ver,' -> ',new_ver]);
      |     %switch - case for specific upgrade information e.g. additional parameter required 
      |     %Change appearance and version information
      |     set_param(gcb,'ForegroundColor',new_color);
      |     set_param(gcb,'tt_iolib_version',new_ver);
      | end
      | %Upgrade Information - standard END
      | catch
      | %Standard catch section BEGIN 
      | disp(' ');
      | disp('------------------------------------------------------------');
      | disp('An error occurred in a callback of the TTC580-BlockLib.');
      | disp('Please copy the following lines and report this to support@tttech.com ');
      | disp('<< begin of error message dump >>');
      | disp(['Version of TTC580-BlockLib: ', get_param(gcb,'tt_iolib_version')]);
      | disp(get_param(gcb,'ttDescription'));
      | disp(gcb);
      | x=lasterror;disp(x.message);
      | disp(get_param(gcb,'MaskValues'));
      | disp(version);
      | disp(computer);
      | disp('<< end of error message dump >>');
      | disp('------------------------------------------------------------');
      | disp(' ');
      | %Standard catch section END
      | end
      mask help:
      | Calculate crc32 for a section out of the EEPROM.
      | In case the given data section exceeds given EEPROM boundaries, non zero ErrorCode is returned.
      mask init:
      | %
      settings: CopyFcn=%deleted
      mask Help: No further help available for this block
      mask Callback EEPROM_mirror: %
      mask Callback iBasicAddr_intern: %
      mask Callback iEndAddr_intern: %
  b_ready : Outport  VectorParamsAs1DForOutWhenUnconnected=off
  wires:
  Compare To Zero1/1 -> Logical Operator/2
  crc32_calc_intern/1(ErrorCode) -> Terminator/1
  Logical Operator/1 -> b_ready/1
  Compare To Zero/1 -> Logical Operator/1
  Memory/1 -> Compare To Zero2/1, crc32_calc_intern/Trigger
  Compare To Zero2/1 -> Write_Mirror/1(b_trigger)
  crc32_calc_intern/2(crc32) -> Write_Mirror/2(data)
  IO_EEPROM_GetStatus/1(ErrorCode) -> IO_EEPROM_Write_ALL/2(GetStatus)
  Write_Mirror/1(ErrorCode_EEPROM_mirror) -> IO_EEPROM_Write_ALL/1(EC_Write_Mirror)
  trigger/1 -> Memory/1
  IO_EEPROM_Write_ALL/1(ErrorCode) -> Compare To Zero/1
  IO_EEPROM_Init/1(ErrorCode) -> EEPROM_Mirror/1(EC_EEPROM_Init)
  IO_EEPROM_GetStatus2/1(ErrorCode) -> Compare To Zero1/1
